simulink model "Cessna"  (R2025b)
settings: Solver=VariableStepAuto  StartTime=0.0  StopTime=100  RelTol=1e-3
settings Model: Creator=joshu  LastModifiedBy=joshu

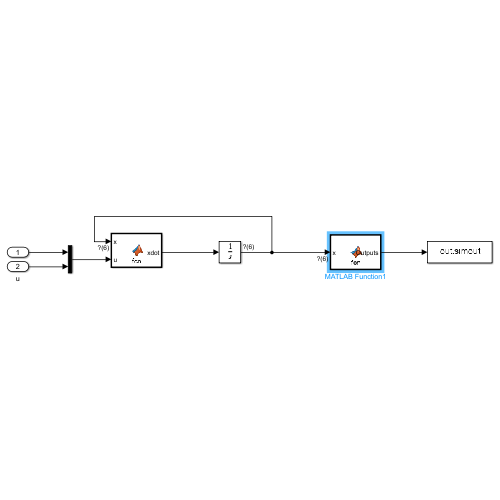
[thumbnail: Simulink's stored preview of the top-level diagram]
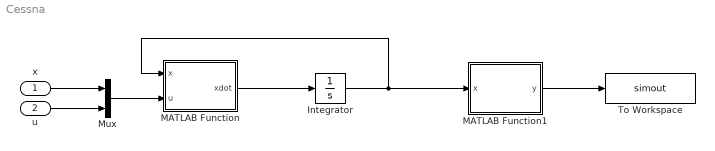
== system Cessna ==
  x : Inport
  u : Inport  Port=2
  Integrator : Integrator  InitialCondition=[200; 5*pi/180; 0; 5*pi/180; 0; 5000]
  MATLAB Function : MATLAB Function  TreatAsAtomicUnit=on
  MATLAB Function1 : MATLAB Function  TreatAsAtomicUnit=on
  Mux : Mux  Inputs=2
  To Workspace : ToWorkspace  VariableName=simout  SaveFormat=Timeseries  SampleTime=-1
  wires:
  x/1 -> Mux/1
  u/1 -> Mux/2
  Mux/1 -> MATLAB Function/2(u)
  MATLAB Function/1(xdot) -> Integrator/1
  Integrator/1 -> MATLAB Function/1(x), MATLAB Function1/1(x)
  MATLAB Function1/1(y) -> To Workspace/1

== matlab function Cessna/MATLAB Function ==
  data: x input; u input; xdot output
function xdot = CessnaEOMs(x,u)
    %% States and Inputs
    V     = x(1);
    alpha = x(2);
    q     = x(3);
    theta = x(4);
    p     = x(5);
    h     = x(6);
    
    el = u(1);
    th = u(2);
    
    %% Cessna Constants
    
    g   = 32.17;
    rho = 0.002377;
    
    W    = 2650;
    S    = 174;
    cbar = 4.9;
    Jz   = 1346;
    m    = W/g;
    
    CL0   = 0.307;
    CLa   = 4.41;
    CL_el = 0.43;
    
    CDM  = 0.0223;
    k    = 0.0554;
    CLDM = 0;
    
    CM_R0  = 0.04;
    CM_Ra  = -0.613;
    CM_Rel = -1.122;
    
    CM_adot = -7.27;
    CM_q    = -12.4;
    CL_adot = 1.7;
    CL_q    = 3.9;
    
    eta = 0.7;
    
    epsilon = 0;
    eT      = 0;
    xcmc = 0;
    
    %% Calculated Variables
    
    gamma = theta - alpha;
    qbar = 0.5*rho*V^2;
    
    % Thrust
    T = (550*th)*eta/max(V,1e-6);
    MT = eT*T;
    
    % Lift
    denL = 1 - qbar*S*(cbar/(2*V))*(CL_adot/(m*V));
    
    numL = qbar*S*( ...
        CL0 + CLa*alpha + CL_el*el ...
      + (cbar/(2*V))*CL_q*q ...
      + (cbar/(2*V))*CL_adot*( q + (W*cos(gamma) - T*sin(alpha - epsilon))/(m*V) ) );
    
    L = numL/denL;
    
    CL = L/(qbar*S);
    
    %alphadot
    alphadot = q + (-L + W*cos(gamma) - T*sin(alpha - epsilon))/(m*V);


    % Drag
    CD = CDM + k*(CL - CLDM)^2;
    D  = qbar*S*CD;
    
    % Momment
    CM = CM_R0 + CM_Ra*alpha + CM_Rel*el ...
       + (cbar/(2*V))*CM_q*q ...
       + (cbar/(2*V))*CM_adot*alphadot ...
       - CL*xcmc;
    
    M = qbar*S*cbar*CM;
    
    %% State Derivatives
    Vdot     = (-D - W*sin(gamma) + T*cos(alpha - epsilon))/m;
    qdot     = (M + MT)/Jz;
    thetadot = q;

    pdot     = V*cos(gamma);
    hdot     = V*sin(gamma);
    
    %% Outputs
    xdot = [Vdot; alphadot; qdot; thetadot; pdot; hdot];

end

== matlab function Cessna/MATLAB Function1 ==
  data: x input; y output
function y = Outputs(x)

    %% States and Inputs
    V     = x(1);
    alpha = rad2deg(x(2));
    q     = x(3);
    theta = rad2deg(x(4));
    p     = x(5);
    h     = x(6);
    
    gamma = theta - alpha;
   
    
    %% Outputs
    y = [V; alpha; gamma; h; p; q];

end
